simulink model "simulink_oscilador_harmonico"  (R2023a)
settings: Solver=FixedStepAuto  StartTime=0.0  StopTime=10.0  FixedStep=1.0e-3  RelTol=1e-3
settings Model: Creator=User  LastModifiedBy=Alexandre
settings SolverCC: AlgebraicLoopSolver=TrustRegion
settings DebuggingCC: UnconnectedInputMsg=warning  UnconnectedOutputMsg=warning  UnconnectedLineMsg=warning
settings ModelReferenceCC: EnableRefExpFcnMdlSchedulingChecks=on
settings RTWCC: DLArmComputeVersion=19.05

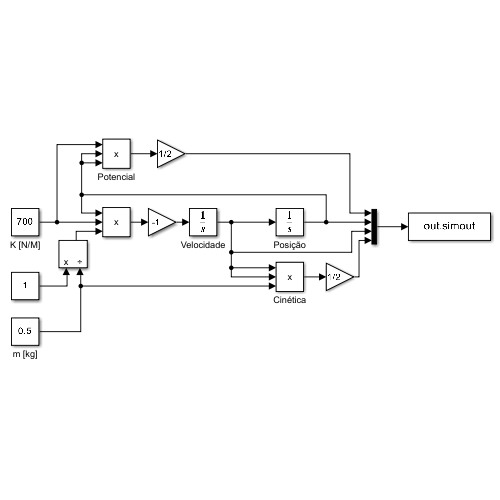
[thumbnail: Simulink's stored preview of the top-level diagram]
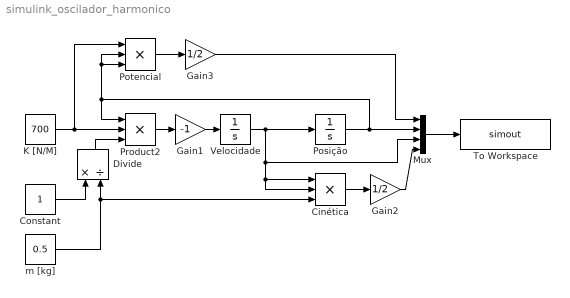
== system simulink_oscilador_harmonico ==
  Cinética : Product  Inputs=3
  Constant : Constant
  Divide : Product  Inputs=*/
  Gain1 : Gain  Gain=-1
  Gain2 : Gain  Gain=1/2
  Gain3 : Gain  Gain=1/2
  K [N/M] : Constant  Value=700
  Mux : Mux
  Posição : Integrator  InitialCondition=0.2
  Potencial : Product  Inputs=3
  Product2 : Product  Inputs=3
  To Workspace : ToWorkspace  VariableName=simout  SampleTime=-1
  Velocidade : Integrator
  m [kg] : Constant  Value=0.5
  wires:
  Posição/1 -> Mux/2, Potencial/2, Potencial/3, Product2/1
  Cinética/1 -> Gain2/1
  Potencial/1 -> Gain3/1
  Mux/1 -> To Workspace/1
  K [N/M]/1 -> Potencial/1, Product2/2
  m [kg]/1 -> Divide/2, Cinética/3
  Product2/1 -> Gain1/1
  Gain1/1 -> Velocidade/1
  Gain3/1 -> Mux/1
  Gain2/1 -> Mux/4
  Velocidade/1 -> Mux/3, Cinética/1, Cinética/2, Posição/1
  Divide/1 -> Product2/3
  Constant/1 -> Divide/1
